simulink model "retificador_bloco_C"  (R2024a)
settings: Solver=FixedStepAuto  StartTime=0.0  StopTime=1.2  FixedStep=5e-6  RelTol=1e-3
InitFcn:
  | clear
  | 
  | Ts = 1/10e3;
  | 
  | v_fase = 120;
  | v_pico = v_fase*sqrt(2);
  | v_linha = v_fase*sqrt(3);
  | v_linha_pico = v_linha*sqrt(2) ;
StopFcn:
  | vdc = out.vdc.signals.values;
  | vdc(1) = vdc(3);
  | vdc(2) = vdc(3);
  | vdc_ref = out.vdc_ref.signals.values*ones(1,length(out.vdc.signals.values))';
  | time = out.vdc.time;
  | 
  | ipq = out.ipq.signals.values;
  | ipq(1) = ipq(3);
  | ipq(2) = ipq(3);
  | ipq_ref = 0*ones(1,length(out.vdc.signals.values))';
  | 
  | t1 = 0.4;
  | t2 = 0.6;
  | t3 = 0.8;
  | t4 = 1.0;
  | t5 = 1.2;
  | 
  | it1 = round((t1*length(time))/time(length(time)));
  | it2 = round((t2*length(time))/time(length(time)));
  | it3 = round((t3*length(time))/time(length(time)));
  | it4 = round((t4*length(time))/time(length(time)));
  | it5 = round((t5*length(time))/time(length(time)));
  | 
  | MAE_vdc = sum(abs(vdc_ref(it1:it5) - vdc(it1:it5)))/length(vdc(it1:it5));
  | MAE_ipq = sum(abs(ipq_ref(it1:it5) - ipq(it1:it5)))/length(ipq(it1:it5));
  | 
  | y_max = max(vdc);
  | figure (1)
  | hold on;
  | plot(time,vdc_ref,'--r','LineWidth',1);
  | plot(time,vdc,'b','LineWidth',1);
  | 
  | str1 = ['MAE_{vdc} = ', num2str(MAE_vdc)];
  | str2 = ['MAE_{ipq} = ', num2str(MAE_ipq)];
  | text(0.01, y_max, str1, 'FontSize', 12, 'Color', 'red');
  | % text(0.01, y_max-1.5, str2, 'FontSize', 12, 'Color', 'red');
  | xlabel('Time [s]')
  | ylabel('DC Voltage [V]')
  | xlim([0 t5]);
  | 
  | 
  | entrada = out.entrada.Data;
  | saida = out.saida.Data;
  | save('dados.mat','entrada','saida');
undefined symbols (not defined in the file or in its folder): Cap, Lfilter, Rfilter
libraries: slpidlib x6, spsAlphaBetaZerotodq0Lib x3, spsdq0toabcLib x3, spsSeriesRLCBranchLib x3, simulink x2, spsIdealSwitchLib x2, SignalEditorBlockLib x2, eeGeneralControl x1, spsThreePhaseSeriesRLCBranchLib x1, spsThreePhaseVIMeasurementLib x1, spsThreePhaseBreakerLib x1, spsThreePhaseSourceLib x1
settings Model: PauseTimes=0.201  Creator=estev  LastModifiedBy=Estevao
settings SFSimCC: SimCustomHeaderCode="#include \"simulink_block.h\""
settings SFSimCC: SimUserSources=|
  | simulink_block.c
  | auxil.c
  | error.c
  | kkt.c
  | lin_alg.c
  | mpc_util.c
  | osqp.c
  | proj.c
  | qdldl.c
  | qdldl_interface.c
  | scaling.c
  | util.c
  | workspace.c
settings SFSimCC: SimUserIncludeDirs=|
  | simulink_c_block02
  | simulink_c_block02/include
  | simulink_c_block02/src/osqp
settings RTWCC: GPUComputeCapability=3.5

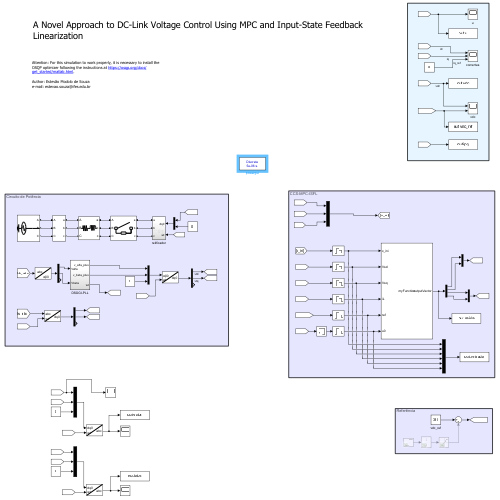
[thumbnail: Simulink's stored preview of the top-level diagram]
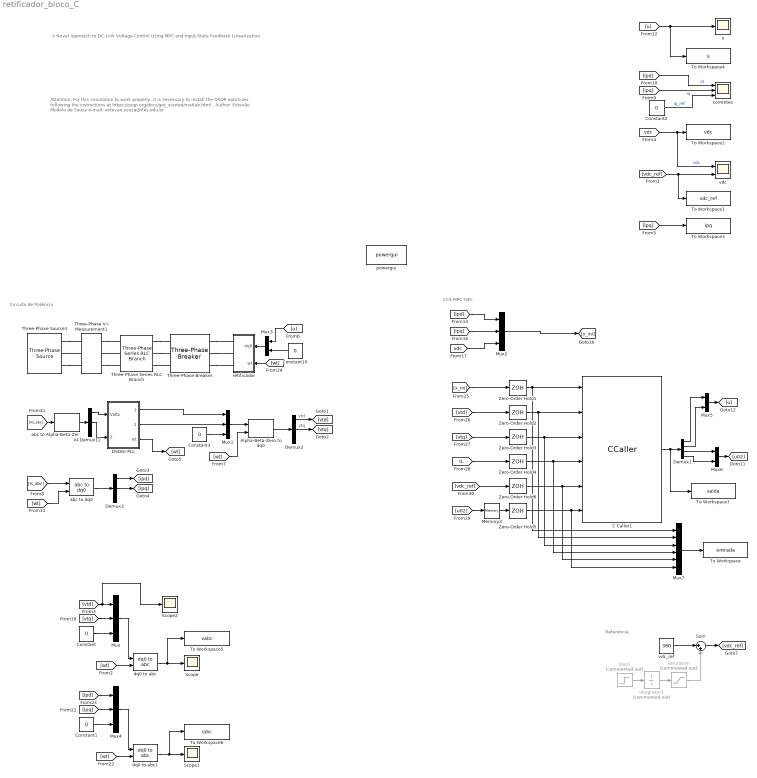
== system retificador_bloco_C ==
  note: Referência
  note: CCS-MPC-ISFL
  note: Attention: For this simulation to work properly, it is necessary to install the OSQP optimizer following the instructions at https://osqp.org/docs/get_started/matlab.html .
      |
      | Author: Estevão Modolo de Souza
      | e-mail: estevao.souza@ifes.edu.br
  note: A Novel Approach to DC-Link Voltage Control Using MPC and Input-State Feedback Linearization
  note: Circuito de Potência
  Alpha-Beta-Zero to dq0 : spsAlphaBetaZerotodq0Lib/Alpha-Beta-Zero to dq0  Alignment=Aligned with phase A axis
  C Caller1 : CCaller  FunctionName=myFunction  PortSpecificationStruct="%)30     .    \" P   8    (     @         %    \"     <    !     0         %  0 \"0    $    _    07)G3F%M90  4&]R=$YA;64 4V-O<&4     26YD97@     5'EP90      4VEZ90      27-';&]B86P   X    X    !@    @    $          4    (     0    4    !         !     %    >%]I;FD    .    .     8    (    !          %    \"     $    %     0         0    !0   'A?:6YI    #@   #@    &    \"     0         !0    @    !  ...(+3771 chars)"  SampleTime=1/10e3
  Constant{,1..3,10} (5 alike) : Constant  Value=0
  DSOGI-PLL : Subsystem
  Demux1 : Demux
  Demux12 : Demux  Outputs=3
  Demux2 : Demux  Outputs=3
  Demux3 : Demux  Outputs=3
  Integrator3 : Integrator  Commented=on
  Memory3 : Memory  InitialCondition=[0;0]
  Mux{,1..2,4} (4 alike) : Mux  Inputs=3
  Mux3 : Mux  Inputs=2
  Mux5 : Mux  Inputs=2
  Mux6 : Mux  Inputs=2
  Mux7 : Mux  Inputs=6
  Saturation : Saturate  Commented=on  UpperLimit=50  LowerLimit=0
  Scope : Scope
  Scope1 : Scope
  Scope2 : Scope
  Step1 : Step  Commented=on  Time=0.5  After=500  SampleTime=0
  Sum : Sum  Inputs=|++
  Three-Phase Series RLC Branch : spsThreePhaseSeriesRLCBranchLib/Three-Phase Series RLC Branch  LConnTagsString=A|B|C  RConnTagsString=A|B|C  BranchType=RL  Resistance=100e-3  Inductance=5e-3  Capacitance=1e-6  Measurements=None
  Three-Phase V-I Measurement1 : spsThreePhaseVIMeasurementLib/Three-Phase V-I Measurement  VoltageMeasurement=phase-to-ground  SetLabelV=on  LabelV=Vs_abc  Vpu=off  VpuLL=off  CurrentMeasurement=yes  SetLabelI=on  LabelI=Is_abc  Ipu=off  Pbase=100e6  Vbase=500e3  OutputType=Complex  PhasorSimulation=off  PSBequivalent=0
  Three-Phase Breaker : spsThreePhaseBreakerLib/Three-Phase Breaker  InitialState=open  SwitchA=on  SwitchB=on  SwitchC=on  SwitchTimes=[0.2]  External=off  BreakerResistance=0.01  SnubberResistance=1e6  SnubberCapacitance=inf  Measurements=None
  Three-Phase Source1 : spsThreePhaseSourceLib/Three-Phase Source  InternalConnection=Yg  VoltagePhases=on  Voltage=220  PhaseAngle=0  Voltage_phases=[120 120 120]  PhaseAngles_phases=[0 -120 +120]  Frequency=50  NonIdealSource=off  SpecifyImpedance=off  Resistance=0.8929  Inductance=16.58e-3  ShortCircuitLevel=100e6  BaseVoltage=25e3  XRratio=7  BusType=swing  Pref=10e3  Qref=0  Prefabc=[10e3, 10e3, 10e3]  Qrefabc=[0, 0, 0]  Qmin=-inf  Qmax=inf
  To Workspace : ToWorkspace  VariableName=entrada  SaveFormat=Timeseries  SampleTime=-1
  To Workspace1 : ToWorkspace  VariableName=vdc_ref  SaveFormat=Structure With Time  SampleTime=-1
  To Workspace2 : ToWorkspace  VariableName=vdc  SaveFormat=Structure With Time  SampleTime=-1
  To Workspace3 : ToWorkspace  VariableName=ipq  SaveFormat=Structure With Time  SampleTime=-1
  To Workspace4 : ToWorkspace  VariableName=u  SaveFormat=Structure With Time  SampleTime=-1
  To Workspace5 : ToWorkspace  VariableName=vabc  SaveFormat=Structure With Time  SampleTime=-1
  To Workspace6 : ToWorkspace  VariableName=iabc  SaveFormat=Structure With Time  SampleTime=-1
  To Workspace7 : ToWorkspace  VariableName=saida  SaveFormat=Timeseries  SampleTime=-1
  Zero-Order Hold{1..6} (6 alike) : ZeroOrderHold  SampleTime=Ts
  abc to Alpha-Beta-Zero1 : spsabctoAlphaBetaZeroLib/abc to Alpha-Beta-Zero
  abc to dq0 : spsabctodq0Lib/abc to dq0  Alignment=Aligned with phase A axis
  correntes : Scope  NumInputPorts=3
  dq0 to abc : spsdq0toabcLib/dq0 to abc  Alignment=Aligned with phase A axis
  dq0 to abc1 : spsdq0toabcLib/dq0 to abc  Alignment=Aligned with phase A axis
  powergui : spspowerguiLib/powergui  Priority=1  SimulationMode=Discrete  SampleTime=5e-6  frequency=60  Iterations=50  frequencyindice=0  Pbase=100e6  ErrMax=1e-4  UnitsV=kV  UnitsW=MW  buscounter=0  FunctionMessages=off  echomessages=off  EnableUseOfTLC=off  CurrentSourceSwitches=off  DisableSnubberDevices=off  DisableRonSwitches=off  DisableVfSwitches=off  DisplayEquations=off  AutomaticDiscreteSolvers=off  SolverType=Tustin/Backward Euler (TBE)  Interpol=off  ExternalGateDelay=off  methode=off  Ts=100  x0status=blocks  SPID=on  SwTol=0  HookPort=off  NonlinearTolerance=1e-4  nMaxIteration=100  ContinueOnMaxIteration=off  RestoreLinks=warning  ResistiveCurrentMeasurement=off  Frange=[0:2:500]  Ylog=off  Xlog=on  ShowGrid=off  save=off  variable=ZData  structure=0  ZoomFFT=off  StartTime=0.0  cycles=1  DisplayStyle=1  fundamental=60  FreqAxis=off  MaxFrequency=1000  frequencyindicesteady=1  RmsSteady=1  display=off
  retificador : Subsystem
  u : Scope
  vdc : Scope  NumInputPorts=2
  vdc_ref : Constant  Value=380
  wires:
  Mux2/1 -> [x_ini]
  Step1/1 -> Integrator3/1
  Integrator3/1 -> Saturation/1
  vdc_ref/1 -> Sum/1
  Saturation/1 -> Sum/2
  [vdc] -> To Workspace2/1, vdc/1  "vdc"
  [ipq] -> To Workspace3/1
  [ipd] -> correntes/1  "id"
  [ipq] -> correntes/2  "iq"
  Constant2/1 -> correntes/3  "iq_ref"
  [u] -> To Workspace4/1, u/1
  [ipd] -> Mux2/1
  [ipq] -> Mux2/2
  [vdc] -> Mux2/3
  Sum/1 -> [vdc_ref]
  [vdc_ref] -> To Workspace1/1, vdc/2
  [wt] -> dq0 to abc/2
  Mux/1 -> dq0 to abc/1
  Constant/1 -> Mux/3
  [vtq] -> Mux/2
  [vtd] -> Scope2/1, Mux/1
  dq0 to abc/1 -> To Workspace5/1, Scope/1
  dq0 to abc1/1 -> To Workspace6/1, Scope1/1
  Constant1/1 -> Mux4/3
  Mux4/1 -> dq0 to abc1/1
  [ipq] -> Mux4/2
  [ipd] -> Mux4/1
  [wt] -> dq0 to abc1/2
  [x_ini] -> Zero-Order Hold1/1
  [vtd] -> Zero-Order Hold2/1
  [vtq] -> Zero-Order Hold3/1
  [iL] -> Zero-Order Hold4/1
  [u02] -> Memory3/1
  Memory3/1 -> Zero-Order Hold5/1
  Zero-Order Hold1/1 -> C Caller1/1, Mux7/1
  Zero-Order Hold2/1 -> C Caller1/2, Mux7/2
  Zero-Order Hold3/1 -> Mux7/3, C Caller1/3
  Zero-Order Hold4/1 -> Mux7/4, C Caller1/4
  Zero-Order Hold5/1 -> Mux7/6, C Caller1/6
  Demux1/2 -> Mux5/2
  Mux5/1 -> [u]
  Demux1/3 -> Mux6/1
  Mux6/1 -> [u02]
  Demux1/4 -> Mux6/2
  Demux1/1 -> Mux5/1
  C Caller1/1 -> To Workspace7/1, Demux1/1
  [vdc_ref] -> Zero-Order Hold6/1
  Zero-Order Hold6/1 -> Mux7/5, C Caller1/5
  [wt] -> Alpha-Beta-Zero to dq0/2
  Demux12/2 -> DSOGI-PLL/2(Vbeta)
  [u] -> Mux3/1
  Constant10/1 -> Mux3/2
  DSOGI-PLL/3(wt) -> [wt]
  Mux3/1 -> retificador/1(dq0)
  DSOGI-PLL/2(v_beta_plus) -> Mux1/2
  [wt] -> retificador/2(wt)
  [wt] -> abc to dq0/2
  Mux1/1 -> Alpha-Beta-Zero to dq0/1
  Demux3/2 -> [ipq]
  [Vs_abc] -> abc to Alpha-Beta-Zero1/1
  abc to Alpha-Beta-Zero1/1 -> Demux12/1
  Demux2/2 -> [vtq]  "vtq"
  Demux2/1 -> [vtd]  "vtd"
  DSOGI-PLL/1(v_alfa_plus) -> Mux1/1
  Demux3/1 -> [ipd]
  Alpha-Beta-Zero to dq0/1 -> Demux2/1
  [Is_abc] -> abc to dq0/1
  Demux12/1 -> DSOGI-PLL/1(Valfa)
  Constant3/1 -> Mux1/3
  abc to dq0/1 -> Demux3/1
  Mux7/1 -> To Workspace/1
  connections:
  Three-Phase Source1/RConn1 -- Three-Phase V-I Measurement1/LConn1
  Three-Phase Source1/RConn3 -- Three-Phase V-I Measurement1/LConn3
  Three-Phase Source1/RConn2 -- Three-Phase V-I Measurement1/LConn2
  Three-Phase Breaker/RConn2 -- retificador/RConn2
  Three-Phase Breaker/RConn3 -- retificador/RConn3
  Three-Phase Series RLC Branch/RConn1 -- Three-Phase Breaker/LConn1
  Three-Phase Series RLC Branch/RConn2 -- Three-Phase Breaker/LConn2
  Three-Phase V-I Measurement1/RConn2 -- Three-Phase Series RLC Branch/LConn2
  Three-Phase Breaker/RConn1 -- retificador/RConn1
  Three-Phase V-I Measurement1/RConn1 -- Three-Phase Series RLC Branch/LConn1
  Three-Phase Breaker/LConn3 -- Three-Phase Series RLC Branch/RConn3
  Three-Phase V-I Measurement1/RConn3 -- Three-Phase Series RLC Branch/LConn3

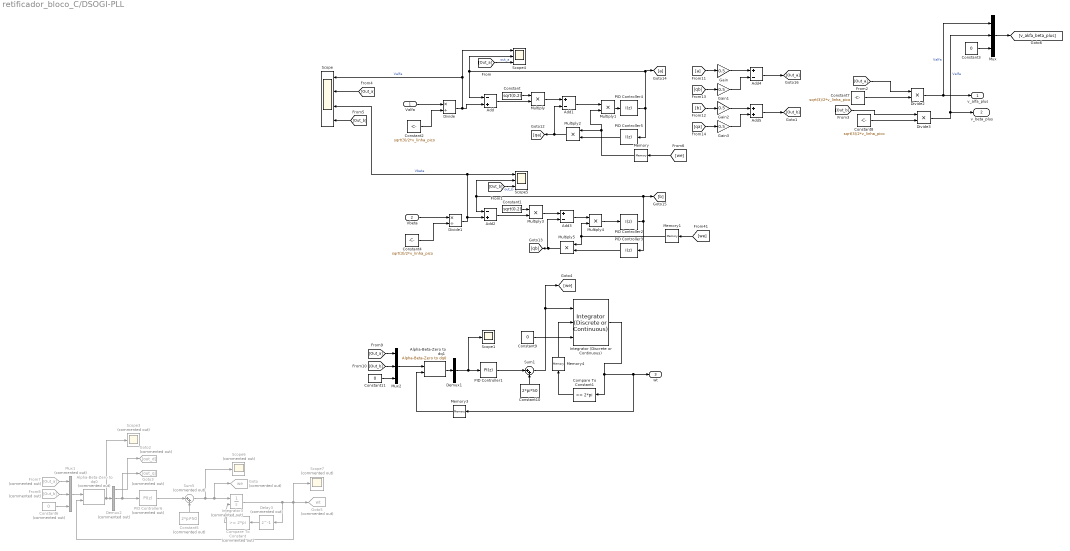
== system retificador_bloco_C/DSOGI-PLL ==
  Valfa : Inport
  Vbeta : Inport  Port=2
  Add : Sum  Inputs=-+
  Add1 : Sum  Inputs=+-
  Add2 : Sum  Inputs=-+
  Add3 : Sum  Inputs=+-
  Add4 : Sum  Inputs=+-
  Add5 : Sum
  Alpha-Beta-Zero to dq0 : spsAlphaBetaZerotodq0Lib/Alpha-Beta-Zero to dq0  Commented=on  Alignment=Aligned with phase A axis
  Alpha-Beta-Zero to dq1 : spsAlphaBetaZerotodq0Lib/Alpha-Beta-Zero to dq0  Alignment=Aligned with phase A axis
  Compare To Constant : simulink/Logic and Bit Operations/Compare To Constant  Commented=on  relop=>=  const=2*pi  OutDataTypeStr=boolean
  Compare To Constant1 : simulink/Logic and Bit Operations/Compare To Constant  relop=>=  const=2*pi  OutDataTypeStr=boolean
  Constant : Constant  Value=sqrt(0.2)
  Constant1 : Constant  Value=sqrt(0.2)
  Constant10 : Constant  Value=2*pi*50
  Constant11 : Constant  Value=0
  Constant{2,4,7..8} (4 alike) : Constant  Value=sqrt(3)/2*v_linha_pico
  Constant3 : Constant  Value=0
  Constant5 : Constant  Commented=on  Value=2*pi*50
  Constant6 : Constant  Commented=on  Value=0
  Constant9 : Constant  Value=0
  Delay3 : Delay  Commented=on  DelayLength=1
  Demux1 : Demux  Outputs=3
  Demux2 : Demux  Commented=on  Outputs=3
  Divide : Product  Inputs=*/
  Divide1 : Product  Inputs=*/
  Divide2 : Product  Inputs=**
  Divide3 : Product  Inputs=**
  From7 : From  Commented=on  GotoTag=Out_a
  From8 : From  Commented=on  GotoTag=Out_b
  Gain{,1..3} (4 alike) : Gain  Gain=0.5
  Goto : Goto  Commented=on  GotoTag=we  TagVisibility=global
  Goto2 : Goto  Commented=on  GotoTag=out_d
  Goto3 : Goto  Commented=on  GotoTag=out_q
  Goto5 : Goto  Commented=on  GotoTag=wt  TagVisibility=global
  Integrator (Discrete or Continuous) : eeGeneralControl/Integrator (Discrete or Continuous)  LabelModeActiveChoice=Discrete  ExternalReset=level  LimitType=Anti-windup  B=inf  A=-inf  Ts=-1
      settings: LibrarySourceBlock=|
      | ee_sl_lib/General Control/Integrator
      | (Discrete or Continuous)
  Integrator3 : Integrator  Commented=on  ExternalReset=either
  Memory : Memory  InitialCondition=2*pi*50
  Memory1 : Memory  InitialCondition=2*pi*50
  Memory3 : Memory  InheritSampleTime=on
  Memory4 : Memory  InheritSampleTime=on
  Multiply{,1..5} (6 alike) : Product
  Mux : Mux  Inputs=3
  Mux1 : Mux  Commented=on  Inputs=3
  Mux2 : Mux  Inputs=3
  PID Controller1 : slpidlib/PID Controller  Controller=PI  Form=Parallel  TimeDomain=Discrete-time  UseExternalTs=off  SampleTime=-1  IntegratorMethod=Forward Euler  FilterMethod=Forward Euler  ControllerParametersSource=internal  P=50  I=50  UseKiTs=off  D=0  UseExternalDerivativeSource=off  N=100  UseFilter=on  TunerSelectOption=Transfer Function Based (PID Tuner App)  InitialConditionSource=internal  InitialConditionForIntegrator=0  InitialConditionForFilter=0  DifferentiatorICPrevScaledInput=0  ExternalReset=none  TrackingMode=off  Kt=1  LimitOutput=off  SatLimitsSource=internal  UpperSaturationLimit=inf  LowerSaturationLimit=-inf  LinearizeAsGain=on  AntiWindupMode=none  Kb=1  LimitIntegrator=off  UpperIntegratorSaturationLimit=inf  LowerIntegratorSaturationLimit=-inf  POutMin=[]  POutMax=[]  IOutMin=[]  IOutMax=[]  DOutMin=[]  DOutMax=[]  NOutMin=[]  NOutMax=[]  SumOutMin=[]  SumOutMax=[]  SaturationOutMin=[]  SaturationOutMax=[]  PParamMin=[]  PParamMax=[]  IParamMin=[]  IParamMax=[]  DParamMin=[]  DParamMax=[]  NParamMin=[]  NParamMax=[]  KbParamMin=[]  KbParamMax=[]  KtParamMin=[]  KtParamMax=[]  KbOutMin=[]  KbOutMax=[]  KtOutMin=[]  KtOutMax=[]  IntegratorOutMin=[]  IntegratorOutMax=[]  FilterOutMin=[]  FilterOutMax=[]  SumI1OutMin=[]  SumI1OutMax=[]  SumI2OutMin=[]  SumI2OutMax=[]  SumI3OutMin=[]  SumI3OutMax=[]  SumI4OutMin=[]  SumI4OutMax=[]  SumDOutMin=[]  SumDOutMax=[]  DifferentiatorOutMin=[]  DifferentiatorOutMax=[]  FilterDiffOutCoefMin=[]  FilterDiffOutCoefMax=[]  ReciprocalOutMin=[]  ReciprocalOutMax=[]  SumDenOutMin=[]  SumDenOutMax=[]  SumNumOutMin=[]  SumNumOutMax=[]  DivideOutMin=[]  DivideOutMax=[]  UdiffTsProdOutMin=[]  UdiffTsProdOutMax=[]  NTsProdOutMin=[]  NTsProdOutMax=[]  UintegralTsProdOutMin=[]  UintegralTsProdOutMax=[]  UngainTsProdOutMin=[]  UngainTsProdOutMax=[]  ClampingZeroOutDataTypeStr=Inherit: Inherit via back propagation  ClampingZeroOutMin=[]  ClampingZeroOutMax=[]  FilterDenConstantOutDataTypeStr=Inherit: Inherit via back propagation  FilterDenConstantOutMin=[]  FilterDenConstantOutMax=[]  PCopyOutDataTypeStr=Inherit: Inherit via back propagation  PCopyOutMin=[]  PCopyOutMax=[]  NCopyOutDataTypeStr=Inherit: Inherit via back propagation  NCopyOutMin=[]  NCopyOutMax=[]  IntegratorContinuousStateAttributes=''  IntegratorStateMustResolveToSignalObject=off  IntegratorRTWStateStorageClass=Auto  FilterContinuousStateAttributes=''  FilterStateMustResolveToSignalObject=off  FilterRTWStateStorageClass=Auto  ParallelPVariant=InternalParameters  IdealPVariant=Disabled  IVariant=InternalParameters  DVariant=Disabled  IntegratorVariant=Discrete  SatVariant=Disabled  AWVariant=Passthrough  PCopyVariant=Disabled  TRVariant=Disabled  FdbkBlocksVariant=Forward  IdealPFdbkVariant=Disabled  SatFdbkVariant=Disabled  DerivativeFilterVariant=Disabled  NVariant=Disabled  NCopyVariant=Disabled_SignalSpec  FilterICVariant=Disabled  IntegratorICVariant=InternalICs  ExternalResetVariant=Disabled  TRSumVariant=Passthrough  SumFdbkVariant=Disabled  SumVariant=Sum_PI  TsampFilterVariant=InternalTs  TsampNgainVariant=Passthrough  TsampIntegralVariant=Disabled_SignalSpec  ExternalSaturationOutDataTypeStr=Inherit: Same as second input  DerivativeSourceVariant=Disabled
  PID Controller2 : slpidlib/PID Controller  Controller=I  Form=Ideal  TimeDomain=Discrete-time  UseExternalTs=off  SampleTime=-1  IntegratorMethod=Forward Euler  FilterMethod=Forward Euler  ControllerParametersSource=internal  P=1  I=1  UseKiTs=off  D=0  UseExternalDerivativeSource=off  N=100  UseFilter=on  TunerSelectOption=Transfer Function Based (PID Tuner App)  InitialConditionSource=internal  InitialConditionForIntegrator=0  InitialConditionForFilter=0  DifferentiatorICPrevScaledInput=0  ExternalReset=none  TrackingMode=off  Kt=1  LimitOutput=off  SatLimitsSource=internal  UpperSaturationLimit=1e9  LowerSaturationLimit=-1e9  LinearizeAsGain=on  AntiWindupMode=none  Kb=1  LimitIntegrator=off  UpperIntegratorSaturationLimit=inf  LowerIntegratorSaturationLimit=-inf  POutMin=[]  POutMax=[]  IOutMin=[]  IOutMax=[]  DOutMin=[]  DOutMax=[]  NOutMin=[]  NOutMax=[]  SumOutMin=[]  SumOutMax=[]  SaturationOutMin=[]  SaturationOutMax=[]  PParamMin=[]  PParamMax=[]  IParamMin=[]  IParamMax=[]  DParamMin=[]  DParamMax=[]  NParamMin=[]  NParamMax=[]  KbParamMin=[]  KbParamMax=[]  KtParamMin=[]  KtParamMax=[]  KbOutMin=[]  KbOutMax=[]  KtOutMin=[]  KtOutMax=[]  IntegratorOutMin=[]  IntegratorOutMax=[]  FilterOutMin=[]  FilterOutMax=[]  SumI1OutMin=[]  SumI1OutMax=[]  SumI2OutMin=[]  SumI2OutMax=[]  SumI3OutMin=[]  SumI3OutMax=[]  SumI4OutMin=[]  SumI4OutMax=[]  SumDOutMin=[]  SumDOutMax=[]  DifferentiatorOutMin=[]  DifferentiatorOutMax=[]  FilterDiffOutCoefMin=[]  FilterDiffOutCoefMax=[]  ReciprocalOutMin=[]  ReciprocalOutMax=[]  SumDenOutMin=[]  SumDenOutMax=[]  SumNumOutMin=[]  SumNumOutMax=[]  DivideOutMin=[]  DivideOutMax=[]  UdiffTsProdOutMin=[]  UdiffTsProdOutMax=[]  NTsProdOutMin=[]  NTsProdOutMax=[]  UintegralTsProdOutMin=[]  UintegralTsProdOutMax=[]  UngainTsProdOutMin=[]  UngainTsProdOutMax=[]  ClampingZeroOutDataTypeStr=Inherit: Inherit via back propagation  ClampingZeroOutMin=[]  ClampingZeroOutMax=[]  FilterDenConstantOutDataTypeStr=Inherit: Inherit via back propagation  FilterDenConstantOutMin=[]  FilterDenConstantOutMax=[]  PCopyOutDataTypeStr=Inherit: Inherit via back propagation  PCopyOutMin=[]  PCopyOutMax=[]  NCopyOutDataTypeStr=Inherit: Inherit via back propagation  NCopyOutMin=[]  NCopyOutMax=[]  IntegratorContinuousStateAttributes=''  IntegratorStateMustResolveToSignalObject=off  IntegratorRTWStateStorageClass=Auto  FilterContinuousStateAttributes=''  FilterStateMustResolveToSignalObject=off  FilterRTWStateStorageClass=Auto  ParallelPVariant=Disabled  IdealPVariant=Disabled  IVariant=InternalParameters  DVariant=Disabled  IntegratorVariant=Discrete  SatVariant=Disabled  AWVariant=Passthrough  PCopyVariant=Disabled  TRVariant=Disabled  FdbkBlocksVariant=Forward  IdealPFdbkVariant=Disabled  SatFdbkVariant=Disabled  DerivativeFilterVariant=Disabled  NVariant=Disabled  NCopyVariant=Disabled_SignalSpec  FilterICVariant=Disabled  IntegratorICVariant=InternalICs  ExternalResetVariant=Disabled  TRSumVariant=Passthrough  SumFdbkVariant=Disabled  SumVariant=Passthrough_I  TsampFilterVariant=InternalTs  TsampNgainVariant=Passthrough  TsampIntegralVariant=Disabled_SignalSpec  ExternalSaturationOutDataTypeStr=Inherit: Same as second input  DerivativeSourceVariant=Disabled
  PID Controller3 : slpidlib/PID Controller  Controller=I  Form=Parallel  TimeDomain=Discrete-time  UseExternalTs=off  SampleTime=-1  IntegratorMethod=Forward Euler  FilterMethod=Forward Euler  ControllerParametersSource=internal  P=1  I=1  UseKiTs=off  D=0  UseExternalDerivativeSource=off  N=100  UseFilter=on  TunerSelectOption=Transfer Function Based (PID Tuner App)  InitialConditionSource=internal  InitialConditionForIntegrator=0  InitialConditionForFilter=0  DifferentiatorICPrevScaledInput=0  ExternalReset=none  TrackingMode=off  Kt=1  LimitOutput=off  SatLimitsSource=internal  UpperSaturationLimit=1e9  LowerSaturationLimit=-1e9  LinearizeAsGain=on  AntiWindupMode=none  Kb=1  LimitIntegrator=off  UpperIntegratorSaturationLimit=inf  LowerIntegratorSaturationLimit=-inf  POutMin=[]  POutMax=[]  IOutMin=[]  IOutMax=[]  DOutMin=[]  DOutMax=[]  NOutMin=[]  NOutMax=[]  SumOutMin=[]  SumOutMax=[]  SaturationOutMin=[]  SaturationOutMax=[]  PParamMin=[]  PParamMax=[]  IParamMin=[]  IParamMax=[]  DParamMin=[]  DParamMax=[]  NParamMin=[]  NParamMax=[]  KbParamMin=[]  KbParamMax=[]  KtParamMin=[]  KtParamMax=[]  KbOutMin=[]  KbOutMax=[]  KtOutMin=[]  KtOutMax=[]  IntegratorOutMin=[]  IntegratorOutMax=[]  FilterOutMin=[]  FilterOutMax=[]  SumI1OutMin=[]  SumI1OutMax=[]  SumI2OutMin=[]  SumI2OutMax=[]  SumI3OutMin=[]  SumI3OutMax=[]  SumI4OutMin=[]  SumI4OutMax=[]  SumDOutMin=[]  SumDOutMax=[]  DifferentiatorOutMin=[]  DifferentiatorOutMax=[]  FilterDiffOutCoefMin=[]  FilterDiffOutCoefMax=[]  ReciprocalOutMin=[]  ReciprocalOutMax=[]  SumDenOutMin=[]  SumDenOutMax=[]  SumNumOutMin=[]  SumNumOutMax=[]  DivideOutMin=[]  DivideOutMax=[]  UdiffTsProdOutMin=[]  UdiffTsProdOutMax=[]  NTsProdOutMin=[]  NTsProdOutMax=[]  UintegralTsProdOutMin=[]  UintegralTsProdOutMax=[]  UngainTsProdOutMin=[]  UngainTsProdOutMax=[]  ClampingZeroOutDataTypeStr=Inherit: Inherit via back propagation  ClampingZeroOutMin=[]  ClampingZeroOutMax=[]  FilterDenConstantOutDataTypeStr=Inherit: Inherit via back propagation  FilterDenConstantOutMin=[]  FilterDenConstantOutMax=[]  PCopyOutDataTypeStr=Inherit: Inherit via back propagation  PCopyOutMin=[]  PCopyOutMax=[]  NCopyOutDataTypeStr=Inherit: Inherit via back propagation  NCopyOutMin=[]  NCopyOutMax=[]  IntegratorContinuousStateAttributes=''  IntegratorStateMustResolveToSignalObject=off  IntegratorRTWStateStorageClass=Auto  FilterContinuousStateAttributes=''  FilterStateMustResolveToSignalObject=off  FilterRTWStateStorageClass=Auto  ParallelPVariant=Disabled  IdealPVariant=Disabled  IVariant=InternalParameters  DVariant=Disabled  IntegratorVariant=Discrete  SatVariant=Disabled  AWVariant=Passthrough  PCopyVariant=Disabled  TRVariant=Disabled  FdbkBlocksVariant=Forward  IdealPFdbkVariant=Disabled  SatFdbkVariant=Disabled  DerivativeFilterVariant=Disabled  NVariant=Disabled  NCopyVariant=Disabled_SignalSpec  FilterICVariant=Disabled  IntegratorICVariant=InternalICs  ExternalResetVariant=Disabled  TRSumVariant=Passthrough  SumFdbkVariant=Disabled  SumVariant=Passthrough_I  TsampFilterVariant=InternalTs  TsampNgainVariant=Passthrough  TsampIntegralVariant=Disabled_SignalSpec  ExternalSaturationOutDataTypeStr=Inherit: Same as second input  DerivativeSourceVariant=Disabled
  PID Controller4 : slpidlib/PID Controller  Controller=I  Form=Ideal  TimeDomain=Discrete-time  UseExternalTs=off  SampleTime=-1  IntegratorMethod=Forward Euler  FilterMethod=Forward Euler  ControllerParametersSource=internal  P=1  I=1  UseKiTs=off  D=0  UseExternalDerivativeSource=off  N=100  UseFilter=on  TunerSelectOption=Transfer Function Based (PID Tuner App)  InitialConditionSource=internal  InitialConditionForIntegrator=0  InitialConditionForFilter=0  DifferentiatorICPrevScaledInput=0  ExternalReset=none  TrackingMode=off  Kt=1  LimitOutput=off  SatLimitsSource=internal  UpperSaturationLimit=1e9  LowerSaturationLimit=-1e9  LinearizeAsGain=on  AntiWindupMode=none  Kb=1  LimitIntegrator=off  UpperIntegratorSaturationLimit=inf  LowerIntegratorSaturationLimit=-inf  POutMin=[]  POutMax=[]  IOutMin=[]  IOutMax=[]  DOutMin=[]  DOutMax=[]  NOutMin=[]  NOutMax=[]  SumOutMin=[]  SumOutMax=[]  SaturationOutMin=[]  SaturationOutMax=[]  PParamMin=[]  PParamMax=[]  IParamMin=[]  IParamMax=[]  DParamMin=[]  DParamMax=[]  NParamMin=[]  NParamMax=[]  KbParamMin=[]  KbParamMax=[]  KtParamMin=[]  KtParamMax=[]  KbOutMin=[]  KbOutMax=[]  KtOutMin=[]  KtOutMax=[]  IntegratorOutMin=[]  IntegratorOutMax=[]  FilterOutMin=[]  FilterOutMax=[]  SumI1OutMin=[]  SumI1OutMax=[]  SumI2OutMin=[]  SumI2OutMax=[]  SumI3OutMin=[]  SumI3OutMax=[]  SumI4OutMin=[]  SumI4OutMax=[]  SumDOutMin=[]  SumDOutMax=[]  DifferentiatorOutMin=[]  DifferentiatorOutMax=[]  FilterDiffOutCoefMin=[]  FilterDiffOutCoefMax=[]  ReciprocalOutMin=[]  ReciprocalOutMax=[]  SumDenOutMin=[]  SumDenOutMax=[]  SumNumOutMin=[]  SumNumOutMax=[]  DivideOutMin=[]  DivideOutMax=[]  UdiffTsProdOutMin=[]  UdiffTsProdOutMax=[]  NTsProdOutMin=[]  NTsProdOutMax=[]  UintegralTsProdOutMin=[]  UintegralTsProdOutMax=[]  UngainTsProdOutMin=[]  UngainTsProdOutMax=[]  ClampingZeroOutDataTypeStr=Inherit: Inherit via back propagation  ClampingZeroOutMin=[]  ClampingZeroOutMax=[]  FilterDenConstantOutDataTypeStr=Inherit: Inherit via back propagation  FilterDenConstantOutMin=[]  FilterDenConstantOutMax=[]  PCopyOutDataTypeStr=Inherit: Inherit via back propagation  PCopyOutMin=[]  PCopyOutMax=[]  NCopyOutDataTypeStr=Inherit: Inherit via back propagation  NCopyOutMin=[]  NCopyOutMax=[]  IntegratorContinuousStateAttributes=''  IntegratorStateMustResolveToSignalObject=off  IntegratorRTWStateStorageClass=Auto  FilterContinuousStateAttributes=''  FilterStateMustResolveToSignalObject=off  FilterRTWStateStorageClass=Auto  ParallelPVariant=Disabled  IdealPVariant=Disabled  IVariant=InternalParameters  DVariant=Disabled  IntegratorVariant=Discrete  SatVariant=Disabled  AWVariant=Passthrough  PCopyVariant=Disabled  TRVariant=Disabled  FdbkBlocksVariant=Forward  IdealPFdbkVariant=Disabled  SatFdbkVariant=Disabled  DerivativeFilterVariant=Disabled  NVariant=Disabled  NCopyVariant=Disabled_SignalSpec  FilterICVariant=Disabled  IntegratorICVariant=InternalICs  ExternalResetVariant=Disabled  TRSumVariant=Passthrough  SumFdbkVariant=Disabled  SumVariant=Passthrough_I  TsampFilterVariant=InternalTs  TsampNgainVariant=Passthrough  TsampIntegralVariant=Disabled_SignalSpec  ExternalSaturationOutDataTypeStr=Inherit: Same as second input  DerivativeSourceVariant=Disabled
  PID Controller5 : slpidlib/PID Controller  Controller=I  Form=Parallel  TimeDomain=Discrete-time  UseExternalTs=off  SampleTime=-1  IntegratorMethod=Forward Euler  FilterMethod=Forward Euler  ControllerParametersSource=internal  P=1  I=1  UseKiTs=off  D=0  UseExternalDerivativeSource=off  N=100  UseFilter=on  TunerSelectOption=Transfer Function Based (PID Tuner App)  InitialConditionSource=internal  InitialConditionForIntegrator=0  InitialConditionForFilter=0  DifferentiatorICPrevScaledInput=0  ExternalReset=none  TrackingMode=off  Kt=1  LimitOutput=off  SatLimitsSource=internal  UpperSaturationLimit=1e9  LowerSaturationLimit=-1e9  LinearizeAsGain=on  AntiWindupMode=none  Kb=1  LimitIntegrator=off  UpperIntegratorSaturationLimit=inf  LowerIntegratorSaturationLimit=-inf  POutMin=[]  POutMax=[]  IOutMin=[]  IOutMax=[]  DOutMin=[]  DOutMax=[]  NOutMin=[]  NOutMax=[]  SumOutMin=[]  SumOutMax=[]  SaturationOutMin=[]  SaturationOutMax=[]  PParamMin=[]  PParamMax=[]  IParamMin=[]  IParamMax=[]  DParamMin=[]  DParamMax=[]  NParamMin=[]  NParamMax=[]  KbParamMin=[]  KbParamMax=[]  KtParamMin=[]  KtParamMax=[]  KbOutMin=[]  KbOutMax=[]  KtOutMin=[]  KtOutMax=[]  IntegratorOutMin=[]  IntegratorOutMax=[]  FilterOutMin=[]  FilterOutMax=[]  SumI1OutMin=[]  SumI1OutMax=[]  SumI2OutMin=[]  SumI2OutMax=[]  SumI3OutMin=[]  SumI3OutMax=[]  SumI4OutMin=[]  SumI4OutMax=[]  SumDOutMin=[]  SumDOutMax=[]  DifferentiatorOutMin=[]  DifferentiatorOutMax=[]  FilterDiffOutCoefMin=[]  FilterDiffOutCoefMax=[]  ReciprocalOutMin=[]  ReciprocalOutMax=[]  SumDenOutMin=[]  SumDenOutMax=[]  SumNumOutMin=[]  SumNumOutMax=[]  DivideOutMin=[]  DivideOutMax=[]  UdiffTsProdOutMin=[]  UdiffTsProdOutMax=[]  NTsProdOutMin=[]  NTsProdOutMax=[]  UintegralTsProdOutMin=[]  UintegralTsProdOutMax=[]  UngainTsProdOutMin=[]  UngainTsProdOutMax=[]  ClampingZeroOutDataTypeStr=Inherit: Inherit via back propagation  ClampingZeroOutMin=[]  ClampingZeroOutMax=[]  FilterDenConstantOutDataTypeStr=Inherit: Inherit via back propagation  FilterDenConstantOutMin=[]  FilterDenConstantOutMax=[]  PCopyOutDataTypeStr=Inherit: Inherit via back propagation  PCopyOutMin=[]  PCopyOutMax=[]  NCopyOutDataTypeStr=Inherit: Inherit via back propagation  NCopyOutMin=[]  NCopyOutMax=[]  IntegratorContinuousStateAttributes=''  IntegratorStateMustResolveToSignalObject=off  IntegratorRTWStateStorageClass=Auto  FilterContinuousStateAttributes=''  FilterStateMustResolveToSignalObject=off  FilterRTWStateStorageClass=Auto  ParallelPVariant=Disabled  IdealPVariant=Disabled  IVariant=InternalParameters  DVariant=Disabled  IntegratorVariant=Discrete  SatVariant=Disabled  AWVariant=Passthrough  PCopyVariant=Disabled  TRVariant=Disabled  FdbkBlocksVariant=Forward  IdealPFdbkVariant=Disabled  SatFdbkVariant=Disabled  DerivativeFilterVariant=Disabled  NVariant=Disabled  NCopyVariant=Disabled_SignalSpec  FilterICVariant=Disabled  IntegratorICVariant=InternalICs  ExternalResetVariant=Disabled  TRSumVariant=Passthrough  SumFdbkVariant=Disabled  SumVariant=Passthrough_I  TsampFilterVariant=InternalTs  TsampNgainVariant=Passthrough  TsampIntegralVariant=Disabled_SignalSpec  ExternalSaturationOutDataTypeStr=Inherit: Same as second input  DerivativeSourceVariant=Disabled
  PID Controller6 : slpidlib/PID Controller  Commented=on  Controller=PI  Form=Parallel  TimeDomain=Discrete-time  UseExternalTs=off  SampleTime=-1  IntegratorMethod=Forward Euler  FilterMethod=Forward Euler  ControllerParametersSource=internal  P=1000  I=1000  UseKiTs=off  D=0  UseExternalDerivativeSource=off  N=100  UseFilter=on  TunerSelectOption=Transfer Function Based (PID Tuner App)  InitialConditionSource=internal  InitialConditionForIntegrator=0  InitialConditionForFilter=0  DifferentiatorICPrevScaledInput=0  ExternalReset=none  TrackingMode=off  Kt=1  LimitOutput=off  SatLimitsSource=internal  UpperSaturationLimit=inf  LowerSaturationLimit=-inf  LinearizeAsGain=on  AntiWindupMode=none  Kb=1  LimitIntegrator=off  UpperIntegratorSaturationLimit=inf  LowerIntegratorSaturationLimit=-inf  POutMin=[]  POutMax=[]  IOutMin=[]  IOutMax=[]  DOutMin=[]  DOutMax=[]  NOutMin=[]  NOutMax=[]  SumOutMin=[]  SumOutMax=[]  SaturationOutMin=[]  SaturationOutMax=[]  PParamMin=[]  PParamMax=[]  IParamMin=[]  IParamMax=[]  DParamMin=[]  DParamMax=[]  NParamMin=[]  NParamMax=[]  KbParamMin=[]  KbParamMax=[]  KtParamMin=[]  KtParamMax=[]  KbOutMin=[]  KbOutMax=[]  KtOutMin=[]  KtOutMax=[]  IntegratorOutMin=[]  IntegratorOutMax=[]  FilterOutMin=[]  FilterOutMax=[]  SumI1OutMin=[]  SumI1OutMax=[]  SumI2OutMin=[]  SumI2OutMax=[]  SumI3OutMin=[]  SumI3OutMax=[]  SumI4OutMin=[]  SumI4OutMax=[]  SumDOutMin=[]  SumDOutMax=[]  DifferentiatorOutMin=[]  DifferentiatorOutMax=[]  FilterDiffOutCoefMin=[]  FilterDiffOutCoefMax=[]  ReciprocalOutMin=[]  ReciprocalOutMax=[]  SumDenOutMin=[]  SumDenOutMax=[]  SumNumOutMin=[]  SumNumOutMax=[]  DivideOutMin=[]  DivideOutMax=[]  UdiffTsProdOutMin=[]  UdiffTsProdOutMax=[]  NTsProdOutMin=[]  NTsProdOutMax=[]  UintegralTsProdOutMin=[]  UintegralTsProdOutMax=[]  UngainTsProdOutMin=[]  UngainTsProdOutMax=[]  ClampingZeroOutDataTypeStr=Inherit: Inherit via back propagation  ClampingZeroOutMin=[]  ClampingZeroOutMax=[]  FilterDenConstantOutDataTypeStr=Inherit: Inherit via back propagation  FilterDenConstantOutMin=[]  FilterDenConstantOutMax=[]  PCopyOutDataTypeStr=Inherit: Inherit via back propagation  PCopyOutMin=[]  PCopyOutMax=[]  NCopyOutDataTypeStr=Inherit: Inherit via back propagation  NCopyOutMin=[]  NCopyOutMax=[]  IntegratorContinuousStateAttributes=''  IntegratorStateMustResolveToSignalObject=off  IntegratorRTWStateStorageClass=Auto  FilterContinuousStateAttributes=''  FilterStateMustResolveToSignalObject=off  FilterRTWStateStorageClass=Auto  ParallelPVariant=InternalParameters  IdealPVariant=Disabled  IVariant=InternalParameters  DVariant=Disabled  IntegratorVariant=Discrete  SatVariant=Disabled  AWVariant=Passthrough  PCopyVariant=Disabled  TRVariant=Disabled  FdbkBlocksVariant=Forward  IdealPFdbkVariant=Disabled  SatFdbkVariant=Disabled  DerivativeFilterVariant=Disabled  NVariant=Disabled  NCopyVariant=Disabled_SignalSpec  FilterICVariant=Disabled  IntegratorICVariant=InternalICs  ExternalResetVariant=Disabled  TRSumVariant=Passthrough  SumFdbkVariant=Disabled  SumVariant=Sum_PI  TsampFilterVariant=InternalTs  TsampNgainVariant=Passthrough  TsampIntegralVariant=Disabled_SignalSpec  ExternalSaturationOutDataTypeStr=Inherit: Same as second input  DerivativeSourceVariant=Disabled
  Scope : Scope  NumInputPorts=4
  Scope1 : Scope
  Scope3 : Scope  Commented=on
  Scope4 : Scope  NumInputPorts=3
  Scope5 : Scope  NumInputPorts=3
  Scope6 : Scope  Commented=on
  Scope7 : Scope  Commented=on
  Sum1 : Sum  Inputs=|++
  Sum5 : Sum  Commented=on  Inputs=|++
  v_alfa_plus : Outport  VectorParamsAs1DForOutWhenUnconnected=off
  v_beta_plus : Outport  Port=2  VectorParamsAs1DForOutWhenUnconnected=off
  wt : Outport  Port=3
  wires:
  Add/1 -> Multiply/2
  [a] -> Gain/1
  Multiply5/1 -> Add3/2, [qb]
  [qb] -> Gain1/1
  [qa] -> Gain3/1
  Gain/1 -> Add4/1
  PID Controller4/1 -> PID Controller5/1, Add/1, Scope4/2, [a]
  Multiply/1 -> Add1/1
  [b] -> Gain2/1
  Constant/1 -> Multiply/1
  Constant1/1 -> Multiply3/1
  Add1/1 -> Multiply1/1
  Gain3/1 -> Add5/2
  Multiply1/1 -> PID Controller4/1
  Gain1/1 -> Add4/2
  Multiply3/1 -> Add3/1
  Multiply4/1 -> PID Controller2/1
  PID Controller3/1 -> Multiply5/2
  Add2/1 -> Multiply3/2
  Gain2/1 -> Add5/1
  Add3/1 -> Multiply4/1
  Add4/1 -> [Out_a]
  Add5/1 -> [Out_b]
  PID Controller2/1 -> PID Controller3/1, [b], Add2/1, Scope5/2
  [Out_a] -> Scope4/3  "out_a"
  [Out_b] -> Scope5/3  "out_b"
  Valfa/1 -> Divide/1
  Divide/1 -> Scope4/1, Scope/1, Add/2  "Valfa"
  Constant2/1 -> Divide/2
  Vbeta/1 -> Divide1/1
  Divide1/1 -> Scope/3, Scope5/1, Add2/2  "Vbeta"
  Constant4/1 -> Divide1/2
  [Out_a] -> Scope/2
  [Out_b] -> Scope/4
  Multiply2/1 -> Add1/2, [qa]
  From7/1 -> Mux1/1
  Alpha-Beta-Zero to dq0/1 -> Scope3/1, Demux2/1
  Demux2/2 -> Goto3/1, PID Controller6/1
  Constant5/1 -> Sum5/2
  Compare To Constant/1 -> Integrator3/2
  Constant6/1 -> Mux1/3
  Integrator3/1 -> Delay3/1, Goto5/1, Alpha-Beta-Zero to dq0/2, Scope7/1
  From8/1 -> Mux1/2
  Sum5/1 -> Scope6/1, Goto/1, Integrator3/1
  Mux1/1 -> Alpha-Beta-Zero to dq0/1
  PID Controller6/1 -> Sum5/1
  PID Controller5/1 -> Multiply2/2
  Constant7/1 -> Divide2/2
  [Out_a] -> Divide2/1
  Divide2/1 -> Mux/1, v_alfa_plus/1  "Valfa"
  Demux2/1 -> Goto2/1
  Constant8/1 -> Divide3/2
  [Out_b] -> Divide3/1
  Divide3/1 -> Mux/2, v_beta_plus/1  "Valfa"
  [we] -> Memory/1
  [we] -> Memory1/1
  Delay3/1 -> Compare To Constant/1
  PID Controller1/1 -> Sum1/1
  Integrator (Discrete or Continuous)/1 -> Compare To Constant1/1, wt/1, Memory3/1
  Memory3/1 -> Alpha-Beta-Zero to dq1/2
  Mux2/1 -> Alpha-Beta-Zero to dq1/1
  Demux1/2 -> Scope1/1, PID Controller1/1
  Memory4/1 -> Integrator (Discrete or Continuous)/2
  Constant9/1 -> Integrator (Discrete or Continuous)/3
  Compare To Constant1/1 -> Memory4/1
  Sum1/1 -> Integrator (Discrete or Continuous)/1, [we]
  Alpha-Beta-Zero to dq1/1 -> Demux1/1
  Constant10/1 -> Sum1/2
  Constant3/1 -> Mux/3
  Mux/1 -> [v_akfa_beta_plus]
  [Out_a] -> Mux2/1
  Constant11/1 -> Mux2/3
  [Out_b] -> Mux2/2
  Memory/1 -> Multiply1/2, Multiply2/1
  Memory1/1 -> Multiply4/2, Multiply5/1

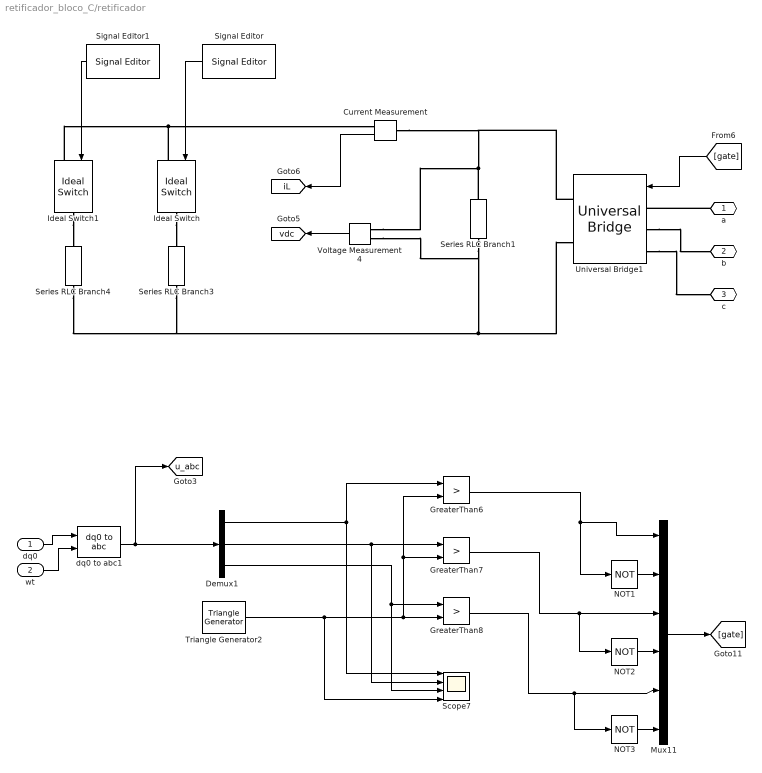
== system retificador_bloco_C/retificador ==
  dq0 : Inport
  wt : Inport  Port=2
  Current Measurement : spsCurrentMeasurementLib/Current Measurement  PhasorSimulation=off  OutputType=Complex  PSBequivalent=0
  Demux1 : Demux  Outputs=3
  GreaterThan6 : RelationalOperator  Operator=>  OutDataTypeStr=boolean  RndMeth=Simplest  InputSameDT=off
  GreaterThan7 : RelationalOperator  Operator=>  OutDataTypeStr=boolean  RndMeth=Simplest  InputSameDT=off
  GreaterThan8 : RelationalOperator  Operator=>  OutDataTypeStr=boolean  RndMeth=Simplest  InputSameDT=off
  Ideal Switch : spsIdealSwitchLib/Ideal Switch  Ron=0.001  Lon=0  IC=0  Rs=1e5  Cs=inf  Measurements=off
  Ideal Switch1 : spsIdealSwitchLib/Ideal Switch  Ron=0.001  Lon=0  IC=0  Rs=1e5  Cs=inf  Measurements=off
  Mux11 : Mux  Inputs=6
  NOT1 : Logic  Operator=NOT  IconShape=distinctive  AllPortsSameDT=off  OutDataTypeStr=boolean
  NOT2 : Logic  Operator=NOT  IconShape=distinctive  AllPortsSameDT=off  OutDataTypeStr=boolean
  NOT3 : Logic  Operator=NOT  IconShape=distinctive  AllPortsSameDT=off  OutDataTypeStr=boolean
  Scope7 : Scope  NumInputPorts=4
  Series RLC Branch1 : spsSeriesRLCBranchLib/Series RLC Branch  LConnTagsString=__new0  RConnTagsString=__new0  BranchType=C  Resistance=Rfilter  Inductance=Lfilter  SetiL0=off  InitialCurrent=0  Capacitance=1000e-6  Setx0=on  InitialVoltage=380  Measurements=None
  Series RLC Branch3 : spsSeriesRLCBranchLib/Series RLC Branch  LConnTagsString=__new0  RConnTagsString=__new0  BranchType=R  Resistance=100  Inductance=Lfilter  SetiL0=off  InitialCurrent=0  Capacitance=Cap  Setx0=on  InitialVoltage=vdc0  Measurements=None
  Series RLC Branch4 : spsSeriesRLCBranchLib/Series RLC Branch  LConnTagsString=__new0  RConnTagsString=__new0  BranchType=R  Resistance=50  Inductance=Lfilter  SetiL0=off  InitialCurrent=0  Capacitance=Cap  Setx0=on  InitialVoltage=vdc0  Measurements=None
  Signal Editor : SignalEditorBlockLib/Signal Editor  FileName=chave01.mat  ActiveScenario=Scenario  ActiveSignal=Signal 1  IsBus=off  OutputBusObjectStr=Bus: BusObject  SampleTime=0  Interpolate=off  ZeroCross=off  OutputAfterFinalValue=Setting to zero  Unit=inherit  PreserveSignalName=on  ApplySigPropsToAllScenarios=on  ApplySigPropsToAllSignals=off
  Signal Editor1 : SignalEditorBlockLib/Signal Editor  FileName=chave02.mat  ActiveScenario=Scenario  ActiveSignal=Signal 1  IsBus=off  OutputBusObjectStr=Bus: BusObject  SampleTime=0  Interpolate=off  ZeroCross=off  OutputAfterFinalValue=Setting to zero  Unit=inherit  PreserveSignalName=on  ApplySigPropsToAllScenarios=on  ApplySigPropsToAllSignals=off
  Triangle Generator2 : spsTriangleGeneratorLib/Triangle Generator  Freq=1/Ts  Phase=90  Ts=0
  Universal Bridge1 : spsUniversalBridgeLib/Universal Bridge  Arms=3  SnubberResistance=1e6  SnubberCapacitance=inf  Device=IGBT / Diodes  Ron=1e-4  Lon=0  ForwardVoltages="[  0  0  ]"  ForwardVoltage=0  GTOparameters=[ 10e-6 , 20e-6 ]  IGBTparameters=[ 1e-6 , 2e-6 ]*0  Measurements=None  Measurements_2=None  converterType=Rectifier
  Voltage Measurement4 : spsVoltageMeasurementLib/Voltage Measurement  PhasorSimulation=off  OutputType=Complex  PSBequivalent=0
  dq0 to abc1 : spsdq0toabcLib/dq0 to abc  Alignment=Aligned with phase A axis
  a : PMIOPort  Side=Right
  b : PMIOPort  Port=2  Side=Right
  c : PMIOPort  Port=3  Side=Right
  tag scope: iL=global, u_abc=global, vdc=global
  wires:
  dq0 to abc1/1 -> [u_abc], Demux1/1
  Demux1/1 -> GreaterThan6/1, Scope7/1
  Demux1/2 -> GreaterThan7/1, Scope7/2
  Triangle Generator2/1 -> GreaterThan8/2, GreaterThan7/2, GreaterThan6/2, Scope7/4
  Demux1/3 -> Scope7/3, GreaterThan8/1
  dq0/1 -> dq0 to abc1/1
  wt/1 -> dq0 to abc1/2
  [gate] -> Universal Bridge1/1
  NOT1/1 -> Mux11/2
  GreaterThan8/1 -> NOT3/1, Mux11/5
  NOT2/1 -> Mux11/4
  GreaterThan7/1 -> NOT2/1, Mux11/3
  Mux11/1 -> [gate]
  NOT3/1 -> Mux11/6
  GreaterThan6/1 -> NOT1/1, Mux11/1
  Voltage Measurement4/1 -> [vdc]
  Current Measurement/1 -> [iL]
  Signal Editor/1 -> Ideal Switch/1
  Signal Editor1/1 -> Ideal Switch1/1
  connections:
  a/RConn1 -- Universal Bridge1/LConn1
  Universal Bridge1/LConn2 -- b/RConn1
  Universal Bridge1/LConn3 -- c/RConn1
  Ideal Switch/LConn1 -- Ideal Switch1/LConn1 -- Current Measurement/RConn1
  Voltage Measurement4/LConn2 -- Series RLC Branch1/RConn1 -- Series RLC Branch4/RConn1 -- Series RLC Branch3/RConn1 -- Universal Bridge1/RConn2
  Series RLC Branch1/LConn1 -- Current Measurement/LConn1 -- Universal Bridge1/RConn1 -- Voltage Measurement4/LConn1
  Ideal Switch/RConn1 -- Series RLC Branch3/LConn1
  Ideal Switch1/RConn1 -- Series RLC Branch4/LConn1
